simulink model "MPC"  (R2024b)
settings: Solver=FixedStepAuto  StartTime=0.0  StopTime=2500  FixedStep=10  RelTol=1e-3
libraries: cstblocks x13, mpclib x13
settings Model: Creator=Gabriel  LastModifiedBy=Gabriel

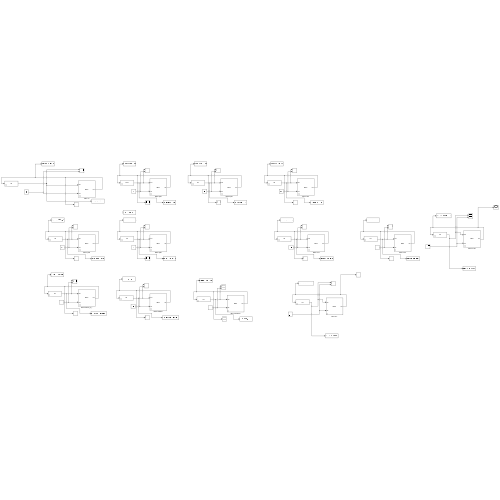
[thumbnail: Simulink's stored preview of the top-level diagram]
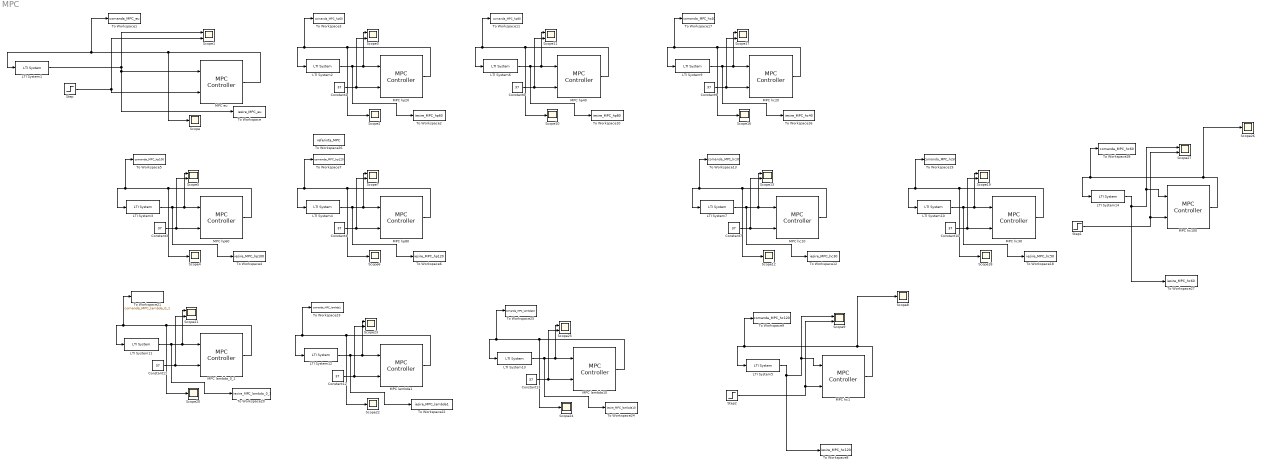
== system MPC ==
  Constant{2..4,6..7,9..13} (10 alike) : Constant  Value=37
  LTI System{1,3..7,9..14} (12 alike) : cstblocks/LTI System  sys=hd  IC=[]  PadeOrder=0
  LTI System2 : cstblocks/LTI System  sys=SYS  IC=[]  PadeOrder=0
  MPC eu : mpclib/MPC Controller  SCDEnableBlockLinearizationSpecification=on  mpcobj=mpcobj  is_multiple=0  enable_value=0  return_u0=off  updateMPCinCallerWorkspace=on  md_inport=off  mv_inport=off  uref_inport=off  return_cost=off  return_mvseq=off  return_qpstatus=off  return_xseq=off  return_state=off  return_ovseq=off  state_inport=off  umin_inport=off  umax_inport=off  ymin_inport=off  ymax_inport=off  cc_inport=off  ywt_inport=off  uwt_inport=off  duwt_inport=off  rhoeps_inport=off  pm_inport=off  MaximumP=10  HorizonChoice=FixedHorizon  n_ts=10  n_p=120  n_mv=1  n_md=0  n_ud=0  n_mo=1  n_uo=0  BlockDataType=double  SampleTimeInherited=off  switch_inport=off
  MPC hc1 : mpclib/MPC Controller  SCDEnableBlockLinearizationSpecification=on  mpcobj=mpc_Hc120  is_multiple=0  enable_value=0  return_u0=off  updateMPCinCallerWorkspace=on  md_inport=off  mv_inport=off  uref_inport=off  return_cost=off  return_mvseq=off  return_qpstatus=off  return_xseq=off  return_state=off  return_ovseq=off  state_inport=off  umin_inport=off  umax_inport=off  ymin_inport=off  ymax_inport=off  cc_inport=off  ywt_inport=off  uwt_inport=off  duwt_inport=off  rhoeps_inport=off  pm_inport=off  MaximumP=10  HorizonChoice=FixedHorizon  n_ts=10  n_p=120  n_mv=1  n_md=0  n_ud=0  n_mo=1  n_uo=0  BlockDataType=double  SampleTimeInherited=off  switch_inport=off
  MPC hc10 : mpclib/MPC Controller  SCDEnableBlockLinearizationSpecification=on  mpcobj=mpc_Hc30  is_multiple=0  enable_value=0  return_u0=off  updateMPCinCallerWorkspace=on  md_inport=off  mv_inport=off  uref_inport=off  return_cost=off  return_mvseq=off  return_qpstatus=off  return_xseq=off  return_state=off  return_ovseq=off  state_inport=off  umin_inport=off  umax_inport=off  ymin_inport=off  ymax_inport=off  cc_inport=off  ywt_inport=off  uwt_inport=off  duwt_inport=off  rhoeps_inport=off  pm_inport=off  MaximumP=10  HorizonChoice=FixedHorizon  n_ts=10  n_p=120  n_mv=1  n_md=0  n_ud=0  n_mo=1  n_uo=0  BlockDataType=double  SampleTimeInherited=off  switch_inport=off
  MPC hc100 : mpclib/MPC Controller  SCDEnableBlockLinearizationSpecification=on  mpcobj=mpc_Hc60  is_multiple=0  enable_value=0  return_u0=off  updateMPCinCallerWorkspace=on  md_inport=off  mv_inport=off  uref_inport=off  return_cost=off  return_mvseq=off  return_qpstatus=off  return_xseq=off  return_state=off  return_ovseq=off  state_inport=off  umin_inport=off  umax_inport=off  ymin_inport=off  ymax_inport=off  cc_inport=off  ywt_inport=off  uwt_inport=off  duwt_inport=off  rhoeps_inport=off  pm_inport=off  MaximumP=10  HorizonChoice=FixedHorizon  n_ts=10  n_p=120  n_mv=1  n_md=0  n_ud=0  n_mo=1  n_uo=0  BlockDataType=double  SampleTimeInherited=off  switch_inport=off
  MPC hc20 : mpclib/MPC Controller  SCDEnableBlockLinearizationSpecification=on  mpcobj=mpc_Hc40  is_multiple=0  enable_value=0  return_u0=off  updateMPCinCallerWorkspace=on  md_inport=off  mv_inport=off  uref_inport=off  return_cost=off  return_mvseq=off  return_qpstatus=off  return_xseq=off  return_state=off  return_ovseq=off  state_inport=off  umin_inport=off  umax_inport=off  ymin_inport=off  ymax_inport=off  cc_inport=off  ywt_inport=off  uwt_inport=off  duwt_inport=off  rhoeps_inport=off  pm_inport=off  MaximumP=10  HorizonChoice=FixedHorizon  n_ts=10  n_p=120  n_mv=1  n_md=0  n_ud=0  n_mo=1  n_uo=0  BlockDataType=double  SampleTimeInherited=off  switch_inport=off
  MPC hc30 : mpclib/MPC Controller  SCDEnableBlockLinearizationSpecification=on  mpcobj=mpc_Hc50  is_multiple=0  enable_value=0  return_u0=off  updateMPCinCallerWorkspace=on  md_inport=off  mv_inport=off  uref_inport=off  return_cost=off  return_mvseq=off  return_qpstatus=off  return_xseq=off  return_state=off  return_ovseq=off  state_inport=off  umin_inport=off  umax_inport=off  ymin_inport=off  ymax_inport=off  cc_inport=off  ywt_inport=off  uwt_inport=off  duwt_inport=off  rhoeps_inport=off  pm_inport=off  MaximumP=10  HorizonChoice=FixedHorizon  n_ts=10  n_p=120  n_mv=1  n_md=0  n_ud=0  n_mo=1  n_uo=0  BlockDataType=double  SampleTimeInherited=off  switch_inport=off
  MPC hp20 : mpclib/MPC Controller  SCDEnableBlockLinearizationSpecification=on  mpcobj=mpc_Hp60  is_multiple=0  enable_value=0  return_u0=off  updateMPCinCallerWorkspace=on  md_inport=off  mv_inport=off  uref_inport=off  return_cost=off  return_mvseq=off  return_qpstatus=off  return_xseq=off  return_state=off  return_ovseq=off  state_inport=off  umin_inport=off  umax_inport=off  ymin_inport=off  ymax_inport=off  cc_inport=off  ywt_inport=off  uwt_inport=off  duwt_inport=off  rhoeps_inport=off  pm_inport=off  MaximumP=10  HorizonChoice=FixedHorizon  n_ts=10  n_p=60  n_mv=1  n_md=0  n_ud=0  n_mo=1  n_uo=0  BlockDataType=double  SampleTimeInherited=off  switch_inport=off
  MPC hp40 : mpclib/MPC Controller  SCDEnableBlockLinearizationSpecification=on  mpcobj=mpc_Hp80  is_multiple=0  enable_value=0  return_u0=off  updateMPCinCallerWorkspace=on  md_inport=off  mv_inport=off  uref_inport=off  return_cost=off  return_mvseq=off  return_qpstatus=off  return_xseq=off  return_state=off  return_ovseq=off  state_inport=off  umin_inport=off  umax_inport=off  ymin_inport=off  ymax_inport=off  cc_inport=off  ywt_inport=off  uwt_inport=off  duwt_inport=off  rhoeps_inport=off  pm_inport=off  MaximumP=10  HorizonChoice=FixedHorizon  n_ts=10  n_p=80  n_mv=1  n_md=0  n_ud=0  n_mo=1  n_uo=0  BlockDataType=double  SampleTimeInherited=off  switch_inport=off
  MPC hp60 : mpclib/MPC Controller  SCDEnableBlockLinearizationSpecification=on  mpcobj=mpc_Hp100  is_multiple=0  enable_value=0  return_u0=off  updateMPCinCallerWorkspace=on  md_inport=off  mv_inport=off  uref_inport=off  return_cost=off  return_mvseq=off  return_qpstatus=off  return_xseq=off  return_state=off  return_ovseq=off  state_inport=off  umin_inport=off  umax_inport=off  ymin_inport=off  ymax_inport=off  cc_inport=off  ywt_inport=off  uwt_inport=off  duwt_inport=off  rhoeps_inport=off  pm_inport=off  MaximumP=10  HorizonChoice=FixedHorizon  n_ts=10  n_p=100  n_mv=1  n_md=0  n_ud=0  n_mo=1  n_uo=0  BlockDataType=double  SampleTimeInherited=off  switch_inport=off
  MPC hp80 : mpclib/MPC Controller  SCDEnableBlockLinearizationSpecification=on  mpcobj=mpc_Hp120  is_multiple=0  enable_value=0  return_u0=off  updateMPCinCallerWorkspace=on  md_inport=off  mv_inport=off  uref_inport=off  return_cost=off  return_mvseq=off  return_qpstatus=off  return_xseq=off  return_state=off  return_ovseq=off  state_inport=off  umin_inport=off  umax_inport=off  ymin_inport=off  ymax_inport=off  cc_inport=off  ywt_inport=off  uwt_inport=off  duwt_inport=off  rhoeps_inport=off  pm_inport=off  MaximumP=10  HorizonChoice=FixedHorizon  n_ts=10  n_p=120  n_mv=1  n_md=0  n_ud=0  n_mo=1  n_uo=0  BlockDataType=double  SampleTimeInherited=off  switch_inport=off
  MPC lambda1 : mpclib/MPC Controller  SCDEnableBlockLinearizationSpecification=on  mpcobj=mpc_lambda_1  is_multiple=0  enable_value=0  return_u0=off  updateMPCinCallerWorkspace=on  md_inport=off  mv_inport=off  uref_inport=off  return_cost=off  return_mvseq=off  return_qpstatus=off  return_xseq=off  return_state=off  return_ovseq=off  state_inport=off  umin_inport=off  umax_inport=off  ymin_inport=off  ymax_inport=off  cc_inport=off  ywt_inport=off  uwt_inport=off  duwt_inport=off  rhoeps_inport=off  pm_inport=off  MaximumP=10  HorizonChoice=FixedHorizon  n_ts=10  n_p=120  n_mv=1  n_md=0  n_ud=0  n_mo=1  n_uo=0  BlockDataType=double  SampleTimeInherited=off  switch_inport=off
  MPC lambda10 : mpclib/MPC Controller  SCDEnableBlockLinearizationSpecification=on  mpcobj=mpc_lambda_10  is_multiple=0  enable_value=0  return_u0=off  updateMPCinCallerWorkspace=on  md_inport=off  mv_inport=off  uref_inport=off  return_cost=off  return_mvseq=off  return_qpstatus=off  return_xseq=off  return_state=off  return_ovseq=off  state_inport=off  umin_inport=off  umax_inport=off  ymin_inport=off  ymax_inport=off  cc_inport=off  ywt_inport=off  uwt_inport=off  duwt_inport=off  rhoeps_inport=off  pm_inport=off  MaximumP=10  HorizonChoice=FixedHorizon  n_ts=10  n_p=120  n_mv=1  n_md=0  n_ud=0  n_mo=1  n_uo=0  BlockDataType=double  SampleTimeInherited=off  switch_inport=off
  MPC lambda_0_1 : mpclib/MPC Controller  SCDEnableBlockLinearizationSpecification=on  mpcobj=mpc_lambda_0_1  is_multiple=0  enable_value=0  return_u0=off  updateMPCinCallerWorkspace=on  md_inport=off  mv_inport=off  uref_inport=off  return_cost=off  return_mvseq=off  return_qpstatus=off  return_xseq=off  return_state=off  return_ovseq=off  state_inport=off  umin_inport=off  umax_inport=off  ymin_inport=off  ymax_inport=off  cc_inport=off  ywt_inport=off  uwt_inport=off  duwt_inport=off  rhoeps_inport=off  pm_inport=off  MaximumP=10  HorizonChoice=FixedHorizon  n_ts=10  n_p=120  n_mv=1  n_md=0  n_ud=0  n_mo=1  n_uo=0  BlockDataType=double  SampleTimeInherited=off  switch_inport=off
  Scope{,2,4,6,8,10,12,16,18,20,22,24,26} (13 alike) : Scope
  Scope{1,3,5,7,9,11,13,17,19,21,23,25,27} (13 alike) : Scope  NumInputPorts=2
  Step : Step  Time=0  After=37  SampleTime=0
  Step1 : Step  Time=0  After=37
  Step2 : Step  Time=0  After=37
  To Workspace : ToWorkspace  VariableName=iesire_MPC_eu  SampleTime=-1
  To Workspace1 : ToWorkspace  VariableName=comanda_MPC_eu  SampleTime=-1
  To Workspace10 : ToWorkspace  VariableName=iesire_MPC_hp80  SampleTime=-1
  To Workspace11 : ToWorkspace  VariableName=comanda_MPC_hp80  SampleTime=-1
  To Workspace12 : ToWorkspace  VariableName=iesire_MPC_hc30  SampleTime=-1
  To Workspace13 : ToWorkspace  VariableName=comanda_MPC_hc30  SampleTime=-1
  To Workspace16 : ToWorkspace  VariableName=iesire_MPC_hc40  SampleTime=-1
  To Workspace17 : ToWorkspace  VariableName=comanda_MPC_hc40  SampleTime=-1
  To Workspace18 : ToWorkspace  VariableName=iesire_MPC_hc50  SampleTime=-1
  To Workspace19 : ToWorkspace  VariableName=comanda_MPC_hc50  SampleTime=-1
  To Workspace2 : ToWorkspace  VariableName=iesire_MPC_hp60  SampleTime=-1
  To Workspace20 : ToWorkspace  VariableName=iesire_MPC_lambda_0_1  SampleTime=-1
  To Workspace21 : ToWorkspace  VariableName=comanda_MPC_lambda_0_1  SampleTime=-1
  To Workspace22 : ToWorkspace  VariableName=iesire_MPC_lambda1  SampleTime=-1
  To Workspace23 : ToWorkspace  VariableName=comanda_MPC_lambda1  SampleTime=-1
  To Workspace24 : ToWorkspace  VariableName=iesire_MPC_lambda10  SampleTime=-1
  To Workspace25 : ToWorkspace  VariableName=comanda_MPC_lambda10  SampleTime=-1
  To Workspace26 : ToWorkspace  VariableName=referinta_MPC  SampleTime=-1
  To Workspace27 : ToWorkspace  VariableName=iesire_MPC_hc60  SampleTime=-1
  To Workspace28 : ToWorkspace  VariableName=comanda_MPC_hc60  SampleTime=-1
  To Workspace3 : ToWorkspace  VariableName=comanda_MPC_hp60  SampleTime=-1
  To Workspace4 : ToWorkspace  VariableName=iesire_MPC_hp100  SampleTime=-1
  To Workspace5 : ToWorkspace  VariableName=comanda_MPC_hp100  SampleTime=-1
  To Workspace6 : ToWorkspace  VariableName=iesire_MPC_hp120  SampleTime=-1
  To Workspace7 : ToWorkspace  VariableName=comanda_MPC_hp120  SampleTime=-1
  To Workspace8 : ToWorkspace  VariableName=iesire_MPC_hc120  SampleTime=-1
  To Workspace9 : ToWorkspace  VariableName=comanda_MPC_hc120  SampleTime=-1
  wires:
  LTI System1/1 -> To Workspace/1, MPC eu/1, Scope1/1
  MPC hp20/1 -> LTI System2/1, To Workspace3/1, Scope2/1
  LTI System2/1 -> Scope3/1, MPC hp20/1, To Workspace2/1
  Constant2/1 -> Scope3/2, MPC hp20/2
  Constant3/1 -> Scope5/2, MPC hp60/2
  LTI System3/1 -> To Workspace4/1, Scope5/1, MPC hp60/1
  MPC hp60/1 -> Scope4/1, To Workspace5/1, LTI System3/1
  MPC hp80/1 -> LTI System4/1, To Workspace7/1, Scope6/1
  LTI System4/1 -> MPC hp80/1, Scope7/1, To Workspace6/1
  Constant4/1 -> MPC hp80/2, Scope7/2
  MPC hp40/1 -> LTI System6/1, To Workspace11/1, Scope10/1
  LTI System6/1 -> MPC hp40/1, Scope11/1, To Workspace10/1
  Constant6/1 -> MPC hp40/2, Scope11/2
  MPC hc10/1 -> LTI System7/1, To Workspace13/1, Scope12/1
  LTI System7/1 -> MPC hc10/1, Scope13/1, To Workspace12/1
  Constant7/1 -> MPC hc10/2, Scope13/2
  MPC hc20/1 -> LTI System9/1, To Workspace17/1, Scope16/1
  LTI System9/1 -> MPC hc20/1, Scope17/1, To Workspace16/1
  Constant9/1 -> MPC hc20/2, Scope17/2
  Constant10/1 -> Scope19/2, MPC hc30/2
  LTI System10/1 -> To Workspace18/1, Scope19/1, MPC hc30/1
  MPC hc30/1 -> Scope18/1, To Workspace19/1, LTI System10/1
  MPC lambda_0_1/1 -> LTI System11/1, To Workspace21/1, Scope20/1
  LTI System11/1 -> MPC lambda_0_1/1, Scope21/1, To Workspace20/1
  Constant11/1 -> MPC lambda_0_1/2, Scope21/2
  Constant12/1 -> Scope23/2, MPC lambda1/2
  LTI System12/1 -> To Workspace22/1, Scope23/1, MPC lambda1/1
  MPC lambda1/1 -> Scope22/1, To Workspace23/1, LTI System12/1
  MPC lambda10/1 -> LTI System13/1, To Workspace25/1, Scope24/1
  LTI System13/1 -> MPC lambda10/1, Scope25/1, To Workspace24/1
  Constant13/1 -> MPC lambda10/2, Scope25/2
  MPC hc100/1 -> LTI System14/1, To Workspace28/1, Scope26/1
  Step1/1 -> MPC hc100/2, Scope27/2
  LTI System14/1 -> Scope27/1, MPC hc100/1, To Workspace27/1
  MPC eu/1 -> Scope/1, To Workspace1/1, LTI System1/1
  Step/1 -> MPC eu/2, Scope1/2
  Step2/1 -> MPC hc1/2, Scope9/2
  LTI System5/1 -> Scope9/1, MPC hc1/1, To Workspace8/1
  MPC hc1/1 -> LTI System5/1, To Workspace9/1, Scope8/1
